simulink model "comparacao_modelo_ensaio"  (R2012b)
settings: Solver=ode45  StartTime=0.0  StopTime=6.2078  FixedStep=5e-5  RelTol=1e-3
undefined symbols (not defined in the file or in its folder): sigbuilder_block
libraries: BLDC x3
settings Model: Creator=h3now  LastModifiedBy=h3now

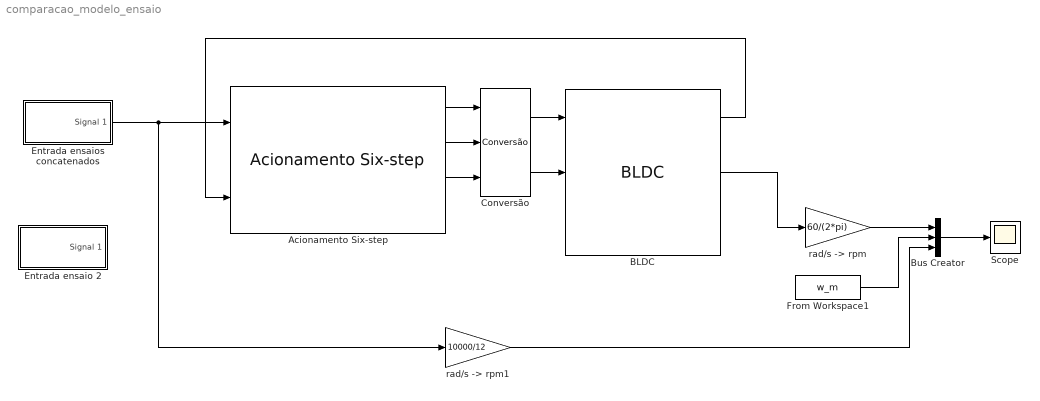
== system comparacao_modelo_ensaio ==
  Acionamento Six-step : BLDC/Acionamento Six-step  P=8
  BLDC : BLDC/BLDC  J=3.84*10^-7  R=23.9/sqrt(3)  L=2.35*10^-3/sqrt(3)  P=8  Kt=11.3*10^-3  Ke=11.3*10^-3  Kd=0  F_stick=0  F_slip=0  default_fcem=on  fcem_a=fcem_a  fcem_b=fcem_b  fcem_c=fcem_c
  Bus Creator : BusCreator  Inputs=3
  Conversão : BLDC/Conversão
  Entrada ensaio 2 : Subsystem  Tag=STV Subsys  LoadFcn=sigbuilder_block('load');  StartFcn=sigbuilder_block('start');  StopFcn=sigbuilder_block('stop');  ClipboardFcn=sigbuilder_block('clipboard');  mask(Sigbuilder block){}
      mask help: Simulink:masks:SigbuilderBlock_MD
      mask init:
      | if ~strcmp(get_param(bdroot(gcbh),'SimulationStatus'),'stopped') tuvar = sigbuilder_block('maskInit'); end
      settings: CopyFcn=sigbuilder_block('copy');  DeleteFcn=sigbuilder_block('delete');  ModelCloseFcn=sigbuilder_block('modelClose');  PreSaveFcn=sigbuilder_block('preSave');  PauseFcn=sigbuilder_block('pause');  ContinueFcn=sigbuilder_block('continue');  NameChangeFcn=sigbuilder_block('namechange');  OpenFcn=sigbuilder_block('open',[0 30 1440 723 ]);  CloseFcn=sigbuilder_block('close');
      mask Display: plot(0, 0, 100, 100,[2, 2, 32, 32, 2], [68, 8, 8, 68, 68],[32, 2], [38, 38], [32, 19, 2],[53, 60, 44], [32, 17, 17, 2],[16, 16, 31, 31]);txt = getActiveGroup(gcbh);text(2, 100, txt,'verticalAlignment', 'top');
  Entrada ensaios concatenados : Subsystem  Tag=STV Subsys  LoadFcn=sigbuilder_block('load');  StartFcn=sigbuilder_block('start');  StopFcn=sigbuilder_block('stop');  ClipboardFcn=sigbuilder_block('clipboard');  mask(Sigbuilder block){}
      mask help: Simulink:masks:SigbuilderBlock_MD
      mask init:
      | if ~strcmp(get_param(bdroot(gcbh),'SimulationStatus'),'stopped') tuvar = sigbuilder_block('maskInit'); end
      settings: CopyFcn=sigbuilder_block('copy');  DeleteFcn=sigbuilder_block('delete');  ModelCloseFcn=sigbuilder_block('modelClose');  PreSaveFcn=sigbuilder_block('preSave');  PauseFcn=sigbuilder_block('pause');  ContinueFcn=sigbuilder_block('continue');  NameChangeFcn=sigbuilder_block('namechange');  OpenFcn=sigbuilder_block('open',[6 28.5 1428 718.5 ]);  CloseFcn=sigbuilder_block('close');
      mask Display: plot(0, 0, 100, 100,[2, 2, 32, 32, 2], [68, 8, 8, 68, 68],[32, 2], [38, 38], [32, 19, 2],[53, 60, 44], [32, 17, 17, 2],[16, 16, 31, 31]);txt = getActiveGroup(gcbh);text(2, 100, txt,'verticalAlignment', 'top');
  From Workspace1 : FromWorkspace  VariableName=w_m  SampleTime=0
  Scope : Scope
      settings: TimeRange=5  YMin=8200  YMax=10000
  "rad/s -> rpm" : Gain  Gain=60/(2*pi)
  "rad/s -> rpm1" : Gain  Gain=10000/12
  wires:
  Acionamento Six-step/1 -> Conversão/1
  Acionamento Six-step/2 -> Conversão/2
  Acionamento Six-step/3 -> Conversão/3
  Conversão/1 -> BLDC/1
  Conversão/2 -> BLDC/2
  BLDC/1 -> Acionamento Six-step/2
  BLDC/2 -> "rad/s -> rpm"/1
  Bus Creator/1 -> Scope/1
  "rad/s -> rpm"/1 -> Bus Creator/1
  Entrada ensaios concatenados/1(Signal 1) -> "rad/s -> rpm1"/1, Acionamento Six-step/1
  From Workspace1/1 -> Bus Creator/2
  "rad/s -> rpm1"/1 -> Bus Creator/3

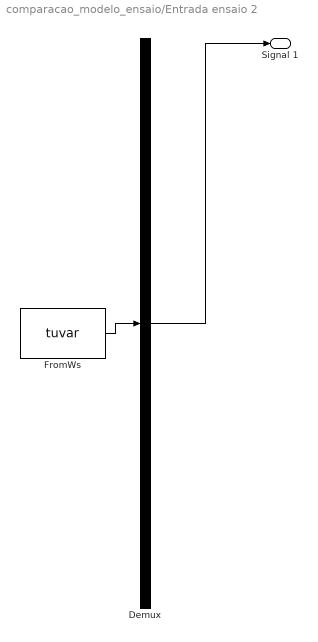
== system comparacao_modelo_ensaio/Entrada ensaio 2 ==
  Demux : Demux  Tag=STV Demux  Outputs=1
  FromWs : FromWorkspace  Tag=STV FromWs  VariableName=tuvar  SampleTime=0
      SigBuilderData=|
      | common.afterFinalStr = 'Extrapolate'
      | common.sampleTime = 0
      | dataSet.timeRange = [0 10]
      | dataSet.name = 'Group 1'
      | sbobj.Groups.Name = 'Group 1'
      | sbobj.Groups.Signals.Name = 'Signal 1'
      | sbobj.Groups.Signals.XData = [0 0.6118 0.6118 1.213 1.213 1.814 1.814 2.419 2.419 10]
      | sbobj.Groups.Signals.YData = [7.2 7.2 8.4 8.4 9.6 9.6 10.8 10.8 12 12]
  Signal 1 : Outport  Tag=STV Outport
  wires:
  Demux/1 -> Signal 1/1
  FromWs/1 -> Demux/1

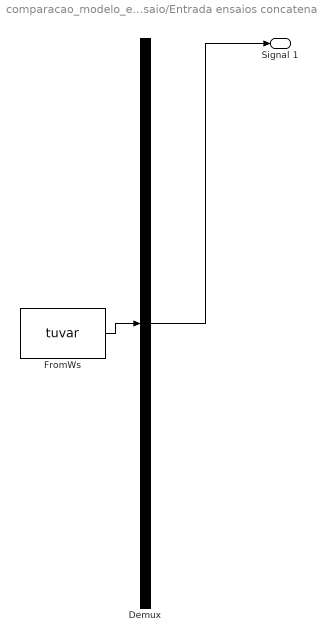
== system comparacao_modelo_ensaio/Entrada ensaios concatenados ==
  Demux : Demux  Tag=STV Demux  Outputs=1
  FromWs : FromWorkspace  Tag=STV FromWs  VariableName=tuvar  SampleTime=0
      SigBuilderData=|
      | common.afterFinalStr = 'Extrapolate'
      | common.sampleTime = 0
      | dataSet.timeRange = [0 10]
      | dataSet.name = 'Group 1'
      | sbobj.Groups.Name = 'Group 1'
      | sbobj.Groups.Signals.Name = 'Signal 1'
      | sbobj.Groups.Signals.XData = [0 0.62 0.62 1.225 1.225 1.811 1.811 2.4 2.4 3.008 3.008 3.61 3.61 4.217 4.217 4.825 4.825 5.415 5.415 9.6 10]
      | sbobj.Groups.Signals.YData = [1.2 1.2 2.4 2.4 3.6 3.6 4.8 4.8 6 6 7.2 7.2 8.4 8.4 9.6 9.6 10.8 10.8 12 12 12]
  Signal 1 : Outport  Tag=STV Outport
  wires:
  Demux/1 -> Signal 1/1
  FromWs/1 -> Demux/1
